simulink model "Practica1_1_modelo"  (R2024a)
settings: Solver=VariableStepAuto  StartTime=0.0  StopTime=10.0  RelTol=1e-3
values from neighbouring files (symbols this model uses):
  op1 = (m2*l2)/(m1 + m2)*l1    (= 0.025)    [Practica 1_1.m]
  op1_2 = 1/l2    (= 4)    [Practica 1_1.m]
  op2 = (m1 + m2)/(m2*l2)    (= 12)    [Practica 1_1.m]
  op2_2 = sin(theta2-theta1)    [Practica 1_1.m]
  op3 = cos(theta2 - theta1)    [Practica 1_1.m]
  op4 = d_theta2 * sin(theta2 - theta1)    [Practica 1_1.m]
  op5 = (g*sin(theta1))/l1    [Practica 1_1.m]
  op_3_2 = g*sin(theta2)    [Practica 1_1.m]
  op_4_2 = 1/l1    (= 3.33333333333)    [Practica 1_1.m]

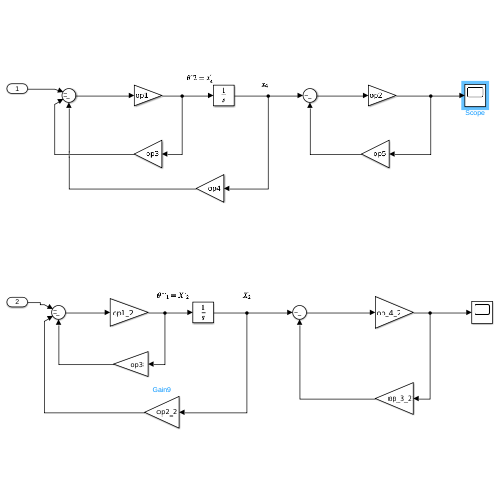
[thumbnail: Simulink's stored preview of the top-level diagram]
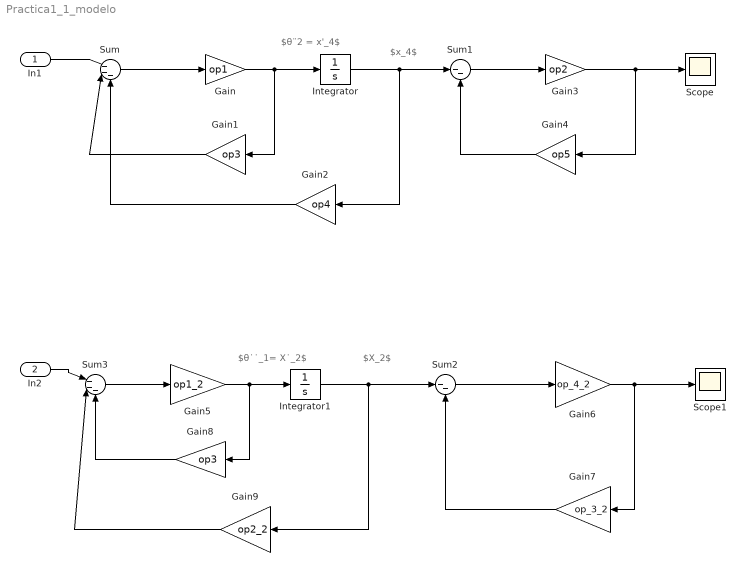
== system Practica1_1_modelo ==
  note: $X_2$
  note: $θ˙˙_1= X˙_2$
  note: $x_4$
  note: $θ¨2 = x'_4$
  In1 : Inport
  In2 : Inport  Port=2
  Gain : Gain  Gain=op1
  Gain1 : Gain  Gain=op3
  Gain2 : Gain  Gain=op4
  Gain3 : Gain  Gain=op2
  Gain4 : Gain  Gain=op5
  Gain5 : Gain  Gain=op1_2
  Gain6 : Gain  Gain=op_4_2
  Gain7 : Gain  Gain=op_3_2
  Gain8 : Gain  Gain=op3
  Gain9 : Gain  Gain=op2_2
  Integrator : Integrator
  Integrator1 : Integrator
  Scope : Scope
  Scope1 : Scope
  Sum : Sum  Inputs=|---
  Sum1 : Sum  Inputs=|--
  Sum2 : Sum  Inputs=|--
  Sum3 : Sum  Inputs=|---
  wires:
  Integrator/1 -> Gain2/1, Sum1/1
  Gain4/1 -> Sum1/2
  Sum1/1 -> Gain3/1
  Gain3/1 -> Scope/1, Gain4/1
  Gain/1 -> Gain1/1, Integrator/1
  Sum/1 -> Gain/1
  Gain1/1 -> Sum/2
  Gain2/1 -> Sum/3
  In1/1 -> Sum/1
  Gain5/1 -> Gain8/1, Integrator1/1
  Integrator1/1 -> Gain9/1, Sum2/1
  Sum2/1 -> Gain6/1
  Gain6/1 -> Scope1/1, Gain7/1
  Gain7/1 -> Sum2/2
  Gain8/1 -> Sum3/3
  Gain9/1 -> Sum3/2
  Sum3/1 -> Gain5/1
  In2/1 -> Sum3/1
